simulink model "ksrbl_4k4t_hdtrig"  (Simulink 6.2)
settings: Solver=ode45  StartTime=0.0  StopTime=20000  RelTol=1e-3
libraries: xbsIndex_r3 x1214, casper_library x120, xps_library x20
(part 21 of 26)

== system ksrbl_4k4t_hdtrig/fft_wideband_real/fft_direct/butterfly2_0/twiddle ==
  a : Inport  Port=1  LatchInput=off
  b : Inport  Port=2  LatchInput=off
  sync : Inport  Port=3  LatchInput=off
  twiddle_general_3mult : casper_library/FFTs/Twiddle/twiddle_general_3mult  Coeffs="[1+0i                     1-0.001534i              1-0.003068i        0.99999-0.0046019i       0.99998-0.0061359i       0.99997-0.0076698i       0.99996-0.0092038i       0.99994-0.010738i        0.99992-0.012272i         0.9999-0.013805i        0.99988-0.015339i        0.99986-0.016873i        0.99983-0.018407i         0.9998-0.01994i         0.99977-0.021474i        0.99974-0.023008i         0.9997-0.024541i        0.99966-0.026075i        0.99962-0.027608i        0.99958-0.029142i        0.99953-0.030675i        0.99948-0.032208i        0.99943-0.033741i        0.99938-0.035274i        0.99932-0.036807i        0.99926-0.03834i          0.9992-0.039873i        0.99914-0.041406i        0.99908-0.042938i        0.99901-0.044471i        0.99894-0.046003i        0.99887-0.047535i         0.9988-0.049068i        0.99872-0.0506i          0.99864-0.052132i        0.99856-0.053664i        0.99848-0.055195i        0.99839-0.056727i         0.9983-0.058258i        0.99821-0.05979i         0.99812-0.061321i        0.99802-0.062852i        0.99793-0.064383i        0.99783-0.065913i        0.99772-0.067444i        0.99762-0.068974i        0.99751-0.070505i         0.9974-0.072035i        0.99729-0.073565i        0.99718-0.075094i        0.99706-0.076624i        0.99694-0.078153i        0.99682-0.079682i         0.9967-0.081211i        0.99657-0.08274i         0.99644-0.084269i        0.99631-0.085797i        0.99618-0.087326i        0.99604-0.088854i        0.99591-0.090381i        0.99577-0.091909i        0.99563-0.093436i        0.99548-0.094963i        0.99533-0.09649i         0.99518-0.098017i        0.99503-0.099544i        0.99488-0.10107i         0.99472-0.1026i          0.99456-0.10412i          0.9944-0.10565i         0.99424-0.10717i         0.99407-0.1087i          0.99391-0.11022i         0.99374-0.11175i         0.99356-0.11327i         0.99339-0.11479i         0.99321-0.11632i         0.99303-0.11784i         0.99285-0.11937i         0.99267-0.12089i         0.99248-0.12241i         0.99229-0.12393i          0.9921-0.12545i         0.99191-0.12698i         0.99171-0.1285i          0.99151-0.13002i         0.99131-0.13154i         0.99111-0.13306i          0.9909-0.13458i          0.9907-0.1361i          0.99049-0.13762i         0.99027-0.13914i         0.99006-0.14066i         0.98984-0.14218i         0.98962-0.1437i           0.9894-0.14521i         0.98918-0.14673i         0.98895-0.14825i         0.98872-0.14976i         0.98849-0.15128i         0.98826-0.1528i          0.98802-0.15431i         0.98778-0.15583i         0.98754-0.15734i          0.9873-0.15886i         0.98706-0.16037i         0.98681-0.16189i         0.98656-0.1634i          0.98631-0.16491i         0.98605-0.16643i          0.9858-0.16794i         0.98554-0.16945i         0.98528-0.17096i         0.98501-0.17247i         0.98475-0.17398i         0.98448-0.17549i         0.98421-0.177i           0.98394-0.17851i         0.98366-0.18002i         0.98339-0.18153i         0.98311-0.18304i         0.98282-0.18455i         0.98254-0.18606i         0.98225-0.18756i         0.98196-0.18907i         0.98167-0.19057i         0.98138-0.19208i         0.98108-0.19359i         0.98079-0.19509i         0.98048-0.19659i         0.98018-0.1981i          0.97988-0.1996i          0.97957-0.2011i          0.97926-0.20261i         0.97895-0.20411i         0.97863-0.20561i         0.97832-0.20711i           0.978-0.20861i         0.97768-0.21011i         0.97735-0.21161i         0.97703-0.21311i          0.9767-0.21461i         0.97637-0.21611i         0.97604-0.2176i           0.9757-0.2191i          0.97536-0.2206i          0.97503-0.22209i         0.97468-0.22359i         0.97434-0.22508i         0.97399-0.22658i         0.97364-0.22807i         0.97329-0.22957i         0.97294-0.23106i         0.97258-0.23255i         0.97223-0.23404i         0.97187-0.23553i          0.9715-0.23702i         0.97114-0.23851i         0.97077-0.24i             0.9704-0.24149i ...(+21586 chars)          ]"  StepPeriod=0  BitWidth=18  add_latency=4  mult_latency=6  bram_latency=4
  a_re : Outport
  a_im : Outport  Port=2
  bw_re : Outport  Port=3
  bw_im : Outport  Port=4
  sync_out : Outport  Port=5
  wires:
  a/1 -> twiddle_general_3mult/1
  b/1 -> twiddle_general_3mult/2
  sync/1 -> twiddle_general_3mult/3
  twiddle_general_3mult/1 -> a_re/1
  twiddle_general_3mult/2 -> a_im/1
  twiddle_general_3mult/3 -> bw_re/1
  twiddle_general_3mult/4 -> bw_im/1
  twiddle_general_3mult/5 -> sync_out/1
